simulink model "Controller"  (R2018b)
settings: configuration reference "control_config" (kept outside this file)
values from neighbouring files (symbols this model uses):
  CONTROL_EXPORT = Simulink.Parameter(CONTROL_EXPORT_VALUE)    [controller_model_init.m]
  CONTROL_PARAM = Simulink.Parameter(CONTROL_PARAM_VALUE)    [controller_model_init.m]
undefined symbols (not defined in the file or in its folder): actuator_cmd, CONTROL_CONST, ControlMode, DiscIntNeverNeededParam, timestamp, VehicleStatus
libraries: simulink x21, FMT_Model_Lib x6
settings Model: Creator=jc  LastModifiedBy=jiachi
settings ConfigSetRef: SourceLocation=Base Workspace

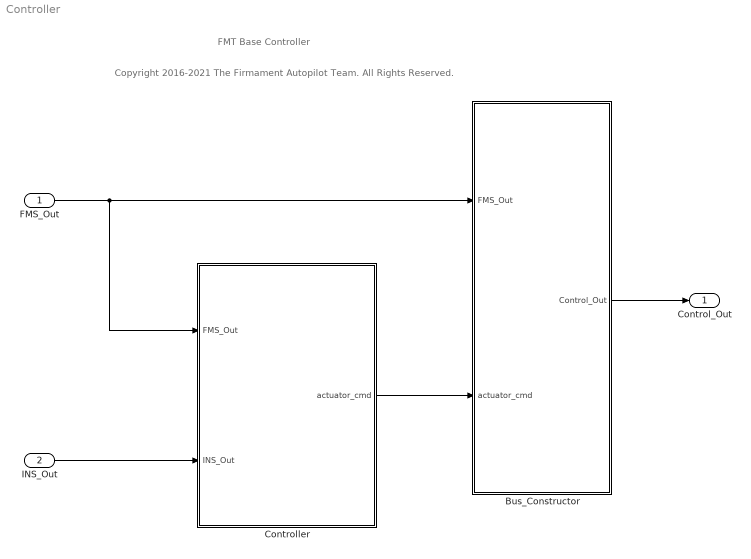
== system Controller ==
  note: Copyright 2016-2021 The Firmament Autopilot Team. All Rights Reserved.
  note: FMT Base Controller
  FMS_Out : Inport  OutDataTypeStr=Bus: FMS_Out_Bus
  INS_Out : Inport  Port=2  OutDataTypeStr=Bus: INS_Out_Bus
  Bus_Constructor : Subsystem
  Controller : Subsystem
  Control_Out : Outport  OutDataTypeStr=Bus: Control_Out_Bus
  wires:
  FMS_Out/1 -> Controller/1(FMS_Out), Bus_Constructor/1(FMS_Out)
  INS_Out/1 -> Controller/2(INS_Out)
  Controller/1(actuator_cmd) -> Bus_Constructor/2(actuator_cmd)
  Bus_Constructor/1(Control_Out) -> Control_Out/1

== system Controller/Bus_Constructor ==
  FMS_Out : Inport
  actuator_cmd : Inport  Port=2
  Bus Assignment : BusAssignment  AssignedSignals=actuator_cmd,timestamp
  Bus Selector : BusSelector  OutputSignals=status
  Bus Selector1 : BusSelector  OutputSignals=actuator_cmd
  Compare To Constant : simulink/Logic and Bit Operations/Compare To Constant  relop===  const=uint8(VehicleStatus.Arm)  OutDataTypeStr=boolean
  Constant : Constant  Value=0  OutDataTypeStr=Bus: Control_Out_Bus
  Switch : Switch  Criteria=u2 > Threshold
  timestamp : Subsystem  mask{sample_time=CONTROL_EXPORT.period}
      mask prompts: sample_time "sample time (ms)"
  Control_Out : Outport
  wires:
  FMS_Out/1 -> Bus Selector1/1, Bus Selector/1
  Bus Selector/1 -> Compare To Constant/1  "<status>"
  Bus Selector1/1 -> Switch/3  "<actuator_cmd>"
  Switch/1 -> Bus Assignment/2
  Compare To Constant/1 -> Switch/2
  actuator_cmd/1 -> Switch/1
  Constant/1 -> Bus Assignment/1
  Bus Assignment/1 -> Control_Out/1
  timestamp/1(timestamp_ms) -> Bus Assignment/3

== system Controller/Controller ==
  FMS_Out : Inport
  INS_Out : Inport  Port=2
  Horizontal_Control : Subsystem
  Static_Control_Allocation : Subsystem
  Vertical_Control : Subsystem
  actuator_cmd : Outport
  wires:
  FMS_Out/1 -> Vertical_Control/1(FMS_Out), Horizontal_Control/1(FMS_Out), Static_Control_Allocation/1(FMS_Out)
  INS_Out/1 -> Horizontal_Control/2(INS_Out), Vertical_Control/2(INS_Out)
  Horizontal_Control/1(rate_dot_cmd_B) -> Static_Control_Allocation/2(rate_dot_cmd_B_normalized)
  Vertical_Control/1(g_force_cmd_B) -> Static_Control_Allocation/3(g_force_cmd_B_normalized)
  Static_Control_Allocation/1(actuator_cmd) -> actuator_cmd/1

== system Controller/Bus_Constructor/timestamp ==
  Constant : Constant  Value=sample_time
  Data Type Conversion : DataTypeConversion  OutDataTypeStr=uint32
  Discrete-Time Integrator : DiscreteIntegrator  IntegratorMethod=Accumulation: Forward Euler  SampleTime=-1  ICPrevOutput=DiscIntNeverNeededParam  ICPrevScaledInput=DiscIntNeverNeededParam
  timestamp_ms : Outport
  wires:
  Discrete-Time Integrator/1 -> Data Type Conversion/1
  Constant/1 -> Discrete-Time Integrator/1
  Data Type Conversion/1 -> timestamp_ms/1

== system Controller/Controller/Horizontal_Control ==
  FMS_Out : Inport
  INS_Out : Inport  Port=2
  Attitude_Controller : Subsystem
  Velocity_Controller : Subsystem
  rate_dot_cmd_B : Outport
  wires:
  Attitude_Controller/1(rate_dot_cmd_B) -> rate_dot_cmd_B/1
  FMS_Out/1 -> Attitude_Controller/2(FMS_Out), Velocity_Controller/1(FMS_Out)
  INS_Out/1 -> Velocity_Controller/2(INS_Out), Attitude_Controller/3(INS_Out)
  Velocity_Controller/1(att_cmd_B_rad) -> Attitude_Controller/1(att_cmd_B_rad)

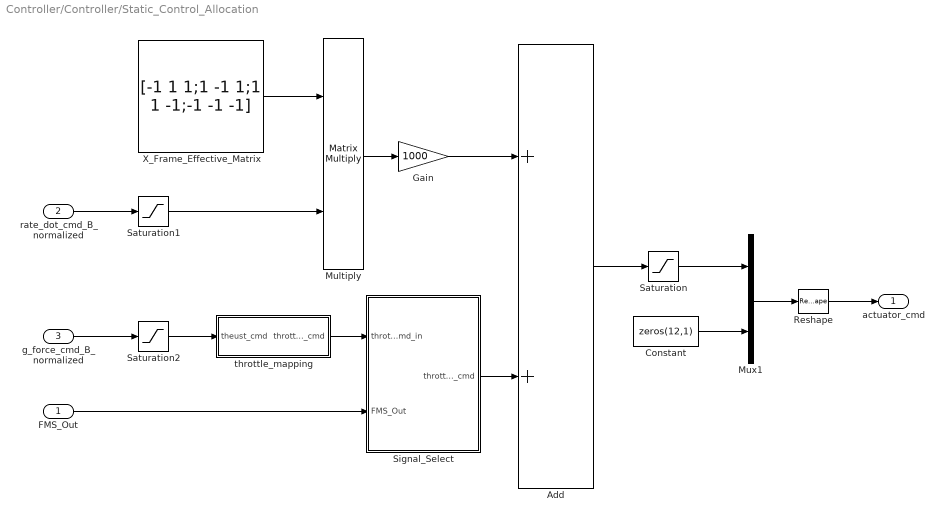
== system Controller/Controller/Static_Control_Allocation ==
  FMS_Out : Inport
  rate_dot_cmd_B_normalized : Inport  Port=2
  g_force_cmd_B_normalized : Inport  Port=3
  Add : Sum  OutDataTypeStr=uint16
  Constant : Constant  Value=zeros(12,1)  VectorParams1D=off  OutDataTypeStr=uint16
  Gain : Gain  Gain=1000  OutDataTypeStr=uint16
  Multiply : Product  Multiplication=Matrix(*)  OutDataTypeStr=Inherit: Same as first input
  Mux1 : Mux  Inputs=2
  Reshape : Reshape  OutputDimensionality=Customize  OutputDimensions=[16,1]
  Saturation : Saturate  UpperLimit=1900  LowerLimit=1100
  Saturation1 : Saturate  UpperLimit=1  LowerLimit=-1
  Saturation2 : Saturate  UpperLimit=1  LowerLimit=-1
  Signal_Select : Subsystem
  X_Frame_Effective_Matrix : Constant  Value=[-1 1 1;1 -1 1;1 1 -1;-1 -1 -1]  OutDataTypeStr=single
  throttle_mapping : Subsystem
  actuator_cmd : Outport
  wires:
  Multiply/1 -> Gain/1
  X_Frame_Effective_Matrix/1 -> Multiply/1
  rate_dot_cmd_B_normalized/1 -> Saturation1/1
  Gain/1 -> Add/1
  g_force_cmd_B_normalized/1 -> Saturation2/1
  Add/1 -> Saturation/1
  Reshape/1 -> actuator_cmd/1
  Mux1/1 -> Reshape/1
  Saturation/1 -> Mux1/1
  Constant/1 -> Mux1/2
  Saturation1/1 -> Multiply/2
  throttle_mapping/1(throttle_cmd) -> Signal_Select/1(throttle_cmd_in)
  Signal_Select/1(throttle_cmd) -> Add/2
  FMS_Out/1 -> Signal_Select/2(FMS_Out)
  Saturation2/1 -> throttle_mapping/1(theust_cmd)

== system Controller/Controller/Vertical_Control ==
  FMS_Out : Inport
  INS_Out : Inport  Port=2
  Veloxity_Z_Controller : Subsystem
  g_force_cmd_B : Outport
  wires:
  INS_Out/1 -> Veloxity_Z_Controller/2(INS_Out)
  Veloxity_Z_Controller/1(g_force_cmd_B) -> g_force_cmd_B/1
  FMS_Out/1 -> Veloxity_Z_Controller/1(FMS_Out)

== system Controller/Controller/Horizontal_Control/Attitude_Controller ==
  att_cmd_B_rad : Inport
  FMS_Out : Inport  Port=2
  INS_Out : Inport  Port=3
  Inner_Loop : Subsystem
  Outter_Loop : Subsystem
  rate_dot_cmd_B : Outport
  wires:
  INS_Out/1 -> Inner_Loop/2(INS_Out), Outter_Loop/2(INS_Out)
  FMS_Out/1 -> Inner_Loop/3(FMS_Out), Outter_Loop/3(FMS_Out)
  att_cmd_B_rad/1 -> Outter_Loop/1(att_cmd_rad)
  Outter_Loop/1(euler_rate_cmd_radPs) -> Inner_Loop/1(euler_rate_cmd_radPs)
  Inner_Loop/1(rate_dot_cmd_B) -> rate_dot_cmd_B/1

== system Controller/Controller/Horizontal_Control/Velocity_Controller ==
  FMS_Out : Inport
  INS_Out : Inport  Port=2
  Accel_to_Attitude_CMD : Subsystem
  Bus Selector : BusSelector  OutputSignals=reset
  Error : Subsystem
  PID_Controller : Subsystem
  Signal_Select : Subsystem
  att_cmd_B_rad : Outport
  wires:
  FMS_Out/1 -> Signal_Select/2(FMS_Out), Error/2(FMS_Out), Bus Selector/1
  PID_Controller/1(accel_cmd_C) -> Signal_Select/1(acc_cmd_in)  "accel_cmd_C_mPs2"
  INS_Out/1 -> Error/1(INS_Out)
  Error/1(uv_err_C_mPs) -> PID_Controller/1(uv_err_C_mPs)
  Accel_to_Attitude_CMD/1(att_cmd_B_rad) -> att_cmd_B_rad/1
  Bus Selector/1 -> PID_Controller/2(reset)  "<reset>"
  Signal_Select/1(acc_cmd_out) -> Accel_to_Attitude_CMD/1(accel_cmd_C_mPs2)

== system Controller/Controller/Static_Control_Allocation/Signal_Select ==
  note: mode:
      | 0: Unknown
      | 1: Mission
      | 2: Position
      | 3: Altitude Hold
      | 4: Manual Mode
      | 5: Acro Mode
  throttle_cmd_in : Inport
  FMS_Out : Inport  Port=2
  Bus Selector1 : BusSelector  OutputSignals=throttle_cmd,ctrl_mode
  Compare To Constant : simulink/Logic and Bit Operations/Compare To Constant  relop===  const=uint8([ControlMode.Manual, ControlMode.Acro, ControlMode.Stabilize])  OutDataTypeStr=boolean
  Compare To Constant1 : simulink/Logic and Bit Operations/Compare To Constant  relop===  const=uint8(ControlMode.Offboard)  OutDataTypeStr=boolean
  Logical Operator : Logic  Operator=OR  Inputs=1  AllPortsSameDT=off  OutDataTypeStr=boolean
  Offboard_Signal_Select : Subsystem
  Switch : Switch  Criteria=u2 > Threshold
  Switch1 : Switch  Criteria=u2 > Threshold
  throttle_cmd : Outport
  wires:
  Compare To Constant/1 -> Logical Operator/1
  FMS_Out/1 -> Offboard_Signal_Select/1(FMS_Out), Bus Selector1/1
  Bus Selector1/1 -> Switch/1  "<throttle_cmd>"
  Bus Selector1/2 -> Compare To Constant1/1, Compare To Constant/1  "<ctrl_mode>"
  Switch/1 -> throttle_cmd/1  "throttle_cmd"
  Logical Operator/1 -> Switch/2
  throttle_cmd_in/1 -> Offboard_Signal_Select/2(throttle_cmd_in), Switch1/3
  Compare To Constant1/1 -> Switch1/2
  Switch1/1 -> Switch/3
  Offboard_Signal_Select/1(throttle_cmd_out) -> Switch1/1

== system Controller/Controller/Static_Control_Allocation/throttle_mapping ==
  theust_cmd : Inport
  Constant1 : Constant  Value=1000  OutDataTypeStr=uint32
  Data Type Conversion : DataTypeConversion  OutDataTypeStr=uint16
  Gain1 : Gain  Gain=1000  OutDataTypeStr=uint32
  Saturation : Saturate  UpperLimit=1  LowerLimit=0
  Sum : Sum  Inputs=|++
  Sum1 : Sum  Inputs=|++
  hover_throttle : Constant  Value=0.5  OutDataTypeStr=Inherit: Inherit via back propagation
  throttle_cmd : Outport
  wires:
  theust_cmd/1 -> Sum/1
  Sum/1 -> Saturation/1
  hover_throttle/1 -> Sum/2
  Gain1/1 -> Sum1/1
  Constant1/1 -> Sum1/2
  Data Type Conversion/1 -> throttle_cmd/1
  Saturation/1 -> Gain1/1
  Sum1/1 -> Data Type Conversion/1

== system Controller/Controller/Vertical_Control/Veloxity_Z_Controller ==
  note: Leave some margin
      | for att control
  FMS_Out : Inport
  INS_Out : Inport  Port=2
  Boosted_Throttle : Subsystem
  Bus Selector : BusSelector  OutputSignals=reset
  Error : Subsystem
  PID_Controller : Subsystem
  Saturation : Saturate  UpperLimit=0.35  LowerLimit=-0.35
  g_force_cmd_B : Outport
  wires:
  Saturation/1 -> g_force_cmd_B/1
  FMS_Out/1 -> Bus Selector/1, Error/1(FMS_Out)
  INS_Out/1 -> Error/2(INS_Out), Boosted_Throttle/2(INS_Out)
  Boosted_Throttle/1(boosted_thrust) -> Saturation/1  "boosted_thrust"
  Error/1(vu_cmd_C_mPs) -> PID_Controller/1(vu_cmd_C_mPs)
  Bus Selector/1 -> PID_Controller/2(reset)  "<reset>"
  PID_Controller/1(thrust_cmd) -> Boosted_Throttle/1(thrust_cmd)

== system Controller/Controller/Horizontal_Control/Attitude_Controller/Inner_Loop ==
  euler_rate_cmd_radPs : Inport
  INS_Out : Inport  Port=2
  FMS_Out : Inport  Port=3
  Bus Selector : BusSelector  OutputSignals=reset
  Rate_Controller : Subsystem
  Signal_Convert : Subsystem
  Signal_Select : Subsystem
  rate_dot_cmd_B : Outport
  wires:
  euler_rate_cmd_radPs/1 -> Signal_Convert/2(euler_rate_cmd)
  Signal_Select/1(out) -> Rate_Controller/1(rate_cmd_radPs)
  Rate_Controller/1(rate_dot_cmd_B) -> rate_dot_cmd_B/1
  Bus Selector/1 -> Rate_Controller/3(reset)  "<reset>"
  INS_Out/1 -> Signal_Convert/3(INS_Out), Rate_Controller/2(INS_Out)
  FMS_Out/1 -> Signal_Convert/1(FMS_Out), Bus Selector/1, Signal_Select/1(FMS_Out)
  Signal_Convert/1(rate_cmd_radPs) -> Signal_Select/2(rate_cmd_radPs)

== system Controller/Controller/Horizontal_Control/Attitude_Controller/Outter_Loop ==
  att_cmd_rad : Inport
  INS_Out : Inport  Port=2
  FMS_Out : Inport  Port=3
  Attitude_Controller : Subsystem
  Signal_Select : Subsystem
  euler_rate_cmd_radPs : Outport
  wires:
  Signal_Select/1(out) -> Attitude_Controller/1(att_cmd_rad)
  FMS_Out/1 -> Signal_Select/2(FMS_Out)
  INS_Out/1 -> Attitude_Controller/2(INS_Out)
  Attitude_Controller/1(euler_rate_cmd_radPs) -> euler_rate_cmd_radPs/1
  att_cmd_rad/1 -> Signal_Select/1(att_cmd_rad)

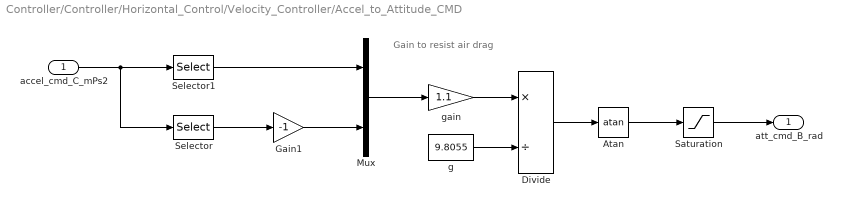
== system Controller/Controller/Horizontal_Control/Velocity_Controller/Accel_to_Attitude_CMD ==
  note: Gain to resist
      | air drag
  accel_cmd_C_mPs2 : Inport
  Atan : Trigonometry  Operator=atan
  Divide : Product  Inputs=*/
  Gain1 : Gain  Gain=-1
  Mux : Mux  Inputs=2
  Saturation : Saturate  UpperLimit=CONTROL_PARAM.ROLL_PITCH_CMD_LIM  LowerLimit=-CONTROL_PARAM.ROLL_PITCH_CMD_LIM
  Selector : Selector  InputPortWidth=2  IndexOptions=Index vector (dialog)  Indices=1  OutputSizes=1
  Selector1 : Selector  InputPortWidth=2  IndexOptions=Index vector (dialog)  Indices=2  OutputSizes=1
  g : Constant  Value=9.8055  OutDataTypeStr=single
  gain : Gain  Gain=1.1
  att_cmd_B_rad : Outport
  wires:
  Mux/1 -> gain/1
  gain/1 -> Divide/1
  Atan/1 -> Saturation/1
  g/1 -> Divide/2
  Divide/1 -> Atan/1
  Selector/1 -> Gain1/1
  Selector1/1 -> Mux/1
  accel_cmd_C_mPs2/1 -> Selector/1, Selector1/1
  Gain1/1 -> Mux/2
  Saturation/1 -> att_cmd_B_rad/1

== system Controller/Controller/Horizontal_Control/Velocity_Controller/Error ==
  INS_Out : Inport
  FMS_Out : Inport  Port=2
  Bus Selector : BusSelector  OutputSignals=u_cmd,v_cmd
  Bus_Select : Subsystem
  Mux : Mux  Inputs=2
  Sum : Sum  Inputs=|+-
  TD : Subsystem
  uv_err_C_mPs : Outport
  wires:
  Sum/1 -> uv_err_C_mPs/1  "uv_error_C_mPs"
  FMS_Out/1 -> Bus Selector/1
  INS_Out/1 -> Bus_Select/1(INS_Out)
  Bus Selector/1 -> Mux/1  "<u_cmd>"
  Bus Selector/2 -> Mux/2  "<v_cmd>"
  Mux/1 -> TD/1(v)
  Bus_Select/1(uv_est_C_mPs) -> Sum/2  "uv_est_C_mPs"
  TD/1(v1) -> Sum/1  "uv_cmd_C_mPs"

== system Controller/Controller/Horizontal_Control/Velocity_Controller/PID_Controller ==
  uv_err_C_mPs : Inport
  reset : Inport  Port=2
  Add : Sum  Inputs=+++
  D_Control : Subsystem  mask{kd=CONTROL_PARAM.VEL_XY_D, max_d=CONTROL_PARAM.VEL_XY_D_MAX, min_d=CONTROL_PARAM.VEL_XY_D_MIN}
  I_Control : Subsystem  mask{ki=CONTROL_PARAM.VEL_XY_I, max_i=CONTROL_PARAM.VEL_XY_I_MAX, min_i=CONTROL_PARAM.VEL_XY_I_MIN}
  P_Control : Subsystem  mask{kp=CONTROL_PARAM.VEL_XY_P}
  accel_cmd_C : Outport
  wires:
  uv_err_C_mPs/1 -> P_Control/1(err), I_Control/1(err), D_Control/1(err)
  reset/1 -> I_Control/2(reset), D_Control/2(reset)
  P_Control/1(p_out) -> Add/1  "accel_p_out"
  I_Control/1(i_out) -> Add/2  "accel_i_out"
  D_Control/1(d_out) -> Add/3  "accel_d_out"
  Add/1 -> accel_cmd_C/1

== system Controller/Controller/Horizontal_Control/Velocity_Controller/Signal_Select ==
  acc_cmd_in : Inport
  FMS_Out : Inport  Port=2
  Bus Selector : BusSelector  OutputSignals=ctrl_mode
  Offboard : simulink/Logic and Bit Operations/Compare To Constant  relop===  const=uint8(ControlMode.Offboard)  OutDataTypeStr=boolean
  Offboard_Signal_Select : Subsystem
  Switch : Switch  Criteria=u2 > Threshold
  acc_cmd_out : Outport
  wires:
  FMS_Out/1 -> Offboard_Signal_Select/1(FMS_Out), Bus Selector/1
  Bus Selector/1 -> Offboard/1  "<ctrl_mode>"
  Offboard/1 -> Switch/2
  Switch/1 -> acc_cmd_out/1
  acc_cmd_in/1 -> Offboard_Signal_Select/2(acc_cmd_in), Switch/3
  Offboard_Signal_Select/1(acc_cmd) -> Switch/1

== system Controller/Controller/Static_Control_Allocation/Signal_Select/Offboard_Signal_Select ==
  FMS_Out : Inport
  throttle_cmd_in : Inport  Port=2
  Bus Selector1 : BusSelector  OutputSignals=cmd_mask
  Bus Selector2 : BusSelector  OutputSignals=throttle_cmd
  Switch : Switch  Criteria=u2 > Threshold
  cmd_throttle valid : simulink/Logic and Bit Operations/Bitwise Operator  logicop=AND  UseBitMask=on  BitMask=bin2dec('1000000000000')  BitMaskRealWorld=Stored Integer
  throttle_cmd_out : Outport
  wires:
  Switch/1 -> throttle_cmd_out/1
  cmd_throttle valid/1 -> Switch/2
  FMS_Out/1 -> Bus Selector2/1, Bus Selector1/1
  Bus Selector1/1 -> cmd_throttle valid/1  "<cmd_mask>"
  Bus Selector2/1 -> Switch/1  "<throttle_cmd>"
  throttle_cmd_in/1 -> Switch/3

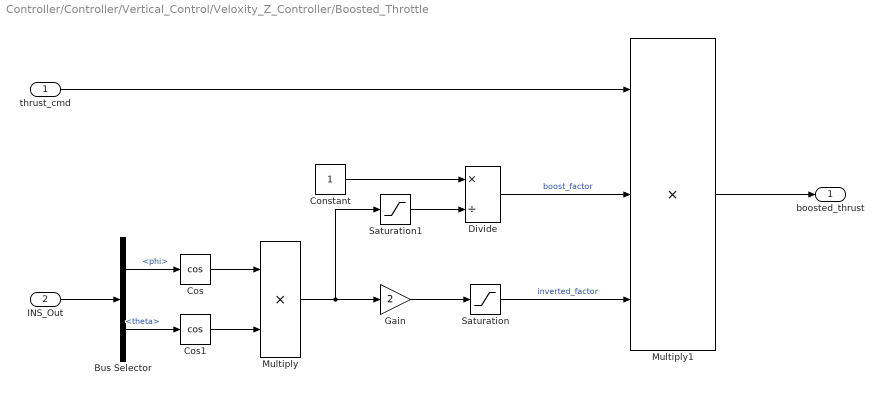
== system Controller/Controller/Vertical_Control/Veloxity_Z_Controller/Boosted_Throttle ==
  thrust_cmd : Inport
  INS_Out : Inport  Port=2
  Bus Selector : BusSelector  OutputSignals=phi,theta
  Constant : Constant  OutDataTypeStr=single
  Cos : Trigonometry  Operator=cos
  Cos1 : Trigonometry  Operator=cos
  Divide : Product  Inputs=*/
  Gain : Gain  Gain=2
  Multiply : Product
  Multiply1 : Product  Inputs=3
  Saturation : Saturate  UpperLimit=1  LowerLimit=0
  Saturation1 : Saturate  UpperLimit=1  LowerLimit=0.5
  boosted_thrust : Outport
  wires:
  INS_Out/1 -> Bus Selector/1
  Bus Selector/1 -> Cos/1  "<phi>"
  Bus Selector/2 -> Cos1/1  "<theta>"
  Cos/1 -> Multiply/1
  Cos1/1 -> Multiply/2
  Multiply/1 -> Saturation1/1, Gain/1
  Gain/1 -> Saturation/1
  Saturation/1 -> Multiply1/3  "inverted_factor"
  Constant/1 -> Divide/1
  Divide/1 -> Multiply1/2  "boost_factor"
  Saturation1/1 -> Divide/2
  thrust_cmd/1 -> Multiply1/1
  Multiply1/1 -> boosted_thrust/1

== system Controller/Controller/Vertical_Control/Veloxity_Z_Controller/Error ==
  FMS_Out : Inport
  INS_Out : Inport  Port=2
  Bus Selector1 : BusSelector  OutputSignals=vd
  Bus Selector2 : BusSelector  OutputSignals=w_cmd
  Gain : Gain  Gain=-1  OutDataTypeStr=Inherit: Same as input
  Signal Copy1 : SignalConversion  OverrideOpt=off
  Sum1 : Sum  Inputs=|+-
  TD : Subsystem
  vu_cmd_C_mPs : Outport
  wires:
  INS_Out/1 -> Bus Selector1/1
  Bus Selector2/1 -> TD/1(v)  "<w_cmd>"
  Bus Selector1/1 -> Signal Copy1/1  "<vd>"
  Gain/1 -> vu_cmd_C_mPs/1
  Sum1/1 -> Gain/1  "w_error_C_mPs"
  FMS_Out/1 -> Bus Selector2/1
  TD/1(v1) -> Sum1/1  "w_cmd_C_mPs"
  Signal Copy1/1 -> Sum1/2  "w_est_C_mPs"

== system Controller/Controller/Vertical_Control/Veloxity_Z_Controller/PID_Controller ==
  vu_cmd_C_mPs : Inport
  reset : Inport  Port=2
  Add : Sum  Inputs=+++
  D_Control : Subsystem  mask{kd=CONTROL_PARAM.VEL_Z_D, max_d=CONTROL_PARAM.VEL_Z_D_MAX, min_d=CONTROL_PARAM.VEL_Z_D_MIN}
  I_Control : Subsystem  mask{ki=CONTROL_PARAM.VEL_Z_I, max_i=CONTROL_PARAM.VEL_Z_I_MAX, min_i=CONTROL_PARAM.VEL_Z_I_MIN}
  P_Control : Subsystem  mask{kp=CONTROL_PARAM.VEL_Z_P}
  thrust_cmd : Outport
  wires:
  P_Control/1(p_out) -> Add/1  "thrust_p_out"
  I_Control/1(i_out) -> Add/2  "thrust_i_out"
  Add/1 -> thrust_cmd/1
  vu_cmd_C_mPs/1 -> D_Control/1(err), I_Control/1(err), P_Control/1(err)
  D_Control/1(d_out) -> Add/3  "thrust_d_out"
  reset/1 -> I_Control/2(reset), D_Control/2(reset)

== system Controller/Controller/Horizontal_Control/Attitude_Controller/Inner_Loop/Rate_Controller ==
  rate_cmd_radPs : Inport
  INS_Out : Inport  Port=2
  reset : Inport  Port=3
  Error : Subsystem
  PID_Controller : Subsystem
  rate_dot_cmd_B : Outport
  wires:
  INS_Out/1 -> Error/2(INS_Out)
  Error/1(rate_err_radPs) -> PID_Controller/1(rate_err_radPs)
  rate_cmd_radPs/1 -> Error/1(rate_cmd_radPs)
  reset/1 -> PID_Controller/2(reset)
  PID_Controller/1(rate_dot_cmd_B) -> rate_dot_cmd_B/1

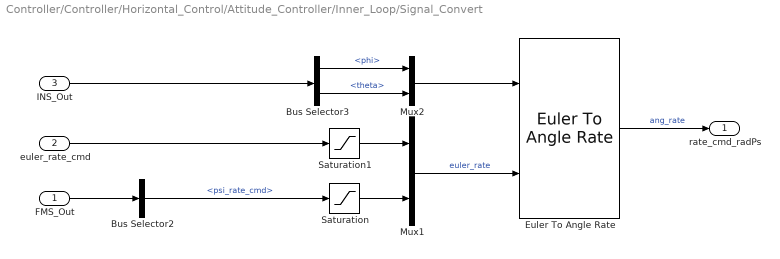
== system Controller/Controller/Horizontal_Control/Attitude_Controller/Inner_Loop/Signal_Convert ==
  FMS_Out : Inport
  euler_rate_cmd : Inport  Port=2
  INS_Out : Inport  Port=3
  Bus Selector2 : BusSelector  OutputSignals=psi_rate_cmd
  Bus Selector3 : BusSelector  OutputSignals=phi,theta
  Euler To Angle Rate : FMT_Model_Lib/Math/Euler To Angle Rate
      settings: SourceProductName=FMT Toolbox
  Mux1 : Mux  Inputs=2
  Mux2 : Mux  Inputs=2
  Saturation : Saturate  UpperLimit=CONTROL_PARAM.R_CMD_LIM  LowerLimit=-CONTROL_PARAM.R_CMD_LIM
  Saturation1 : Saturate  UpperLimit=CONTROL_PARAM.P_Q_CMD_LIM  LowerLimit=-CONTROL_PARAM.P_Q_CMD_LIM
  rate_cmd_radPs : Outport
  wires:
  Bus Selector3/1 -> Mux2/1  "<phi>"
  Mux2/1 -> Euler To Angle Rate/1
  Bus Selector3/2 -> Mux2/2  "<theta>"
  euler_rate_cmd/1 -> Saturation1/1
  Bus Selector2/1 -> Saturation/1  "<psi_rate_cmd>"
  Mux1/1 -> Euler To Angle Rate/2  "euler_rate"
  FMS_Out/1 -> Bus Selector2/1
  INS_Out/1 -> Bus Selector3/1
  Euler To Angle Rate/1 -> rate_cmd_radPs/1  "ang_rate"
  Saturation/1 -> Mux1/2
  Saturation1/1 -> Mux1/1

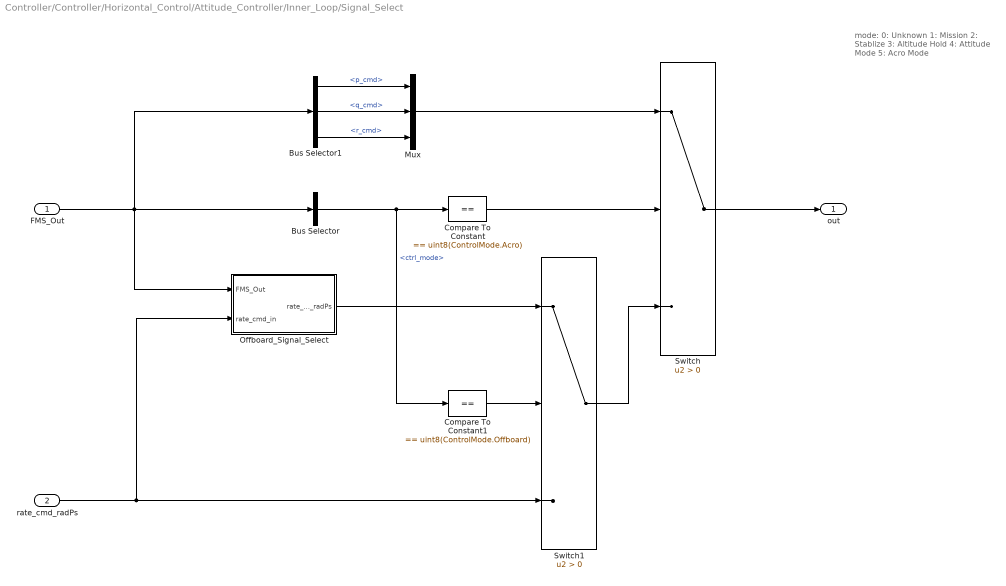
== system Controller/Controller/Horizontal_Control/Attitude_Controller/Inner_Loop/Signal_Select ==
  note: mode:
      | 0: Unknown
      | 1: Mission
      | 2: Stablize
      | 3: Altitude Hold
      | 4: Attitude Mode
      | 5: Acro Mode
  FMS_Out : Inport
  rate_cmd_radPs : Inport  Port=2
  Bus Selector : BusSelector  OutputSignals=ctrl_mode
  Bus Selector1 : BusSelector  OutputSignals=p_cmd,q_cmd,r_cmd
  Compare To Constant : simulink/Logic and Bit Operations/Compare To Constant  relop===  const=uint8(ControlMode.Acro)  OutDataTypeStr=boolean
  Compare To Constant1 : simulink/Logic and Bit Operations/Compare To Constant  relop===  const=uint8(ControlMode.Offboard)  OutDataTypeStr=boolean
  Mux : Mux  Inputs=3
  Offboard_Signal_Select : Subsystem
  Switch : Switch  Criteria=u2 > Threshold
  Switch1 : Switch  Criteria=u2 > Threshold
  out : Outport
  wires:
  FMS_Out/1 -> Bus Selector/1, Offboard_Signal_Select/1(FMS_Out), Bus Selector1/1
  Switch/1 -> out/1
  Bus Selector/1 -> Compare To Constant1/1, Compare To Constant/1  "<ctrl_mode>"
  Compare To Constant/1 -> Switch/2
  Bus Selector1/1 -> Mux/1  "<p_cmd>"
  Bus Selector1/2 -> Mux/2  "<q_cmd>"
  Bus Selector1/3 -> Mux/3  "<r_cmd>"
  Mux/1 -> Switch/1
  rate_cmd_radPs/1 -> Switch1/3, Offboard_Signal_Select/2(rate_cmd_in)
  Switch1/1 -> Switch/3
  Offboard_Signal_Select/1(rate_cmd_radPs) -> Switch1/1
  Compare To Constant1/1 -> Switch1/2

== system Controller/Controller/Horizontal_Control/Attitude_Controller/Outter_Loop/Attitude_Controller ==
  att_cmd_rad : Inport
  INS_Out : Inport  Port=2
  Error : Subsystem
  Sqrt_Root_Controller : Subsystem
  euler_rate_cmd_radPs : Outport
  wires:
  INS_Out/1 -> Error/2(INS_Out)
  Sqrt_Root_Controller/1(euler_rate_cmd_radPs) -> euler_rate_cmd_radPs/1
  att_cmd_rad/1 -> Error/1(att_cmd)
  Error/1(euler_err_rad) -> Sqrt_Root_Controller/1(euler_err_rad)

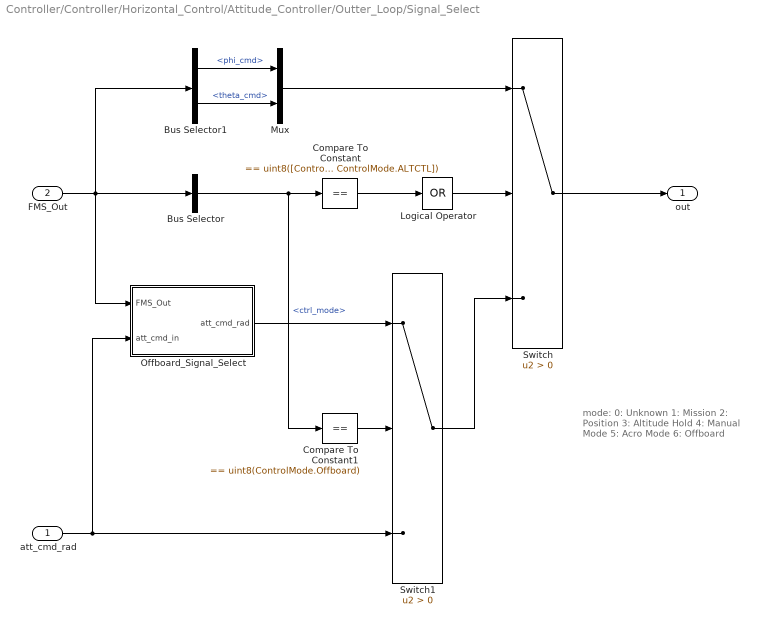
== system Controller/Controller/Horizontal_Control/Attitude_Controller/Outter_Loop/Signal_Select ==
  note: mode:
      | 0: Unknown
      | 1: Mission
      | 2: Position
      | 3: Altitude Hold
      | 4: Manual Mode
      | 5: Acro Mode
      | 6: Offboard
  att_cmd_rad : Inport
  FMS_Out : Inport  Port=2
  Bus Selector : BusSelector  OutputSignals=ctrl_mode
  Bus Selector1 : BusSelector  OutputSignals=phi_cmd,theta_cmd
  Compare To Constant : simulink/Logic and Bit Operations/Compare To Constant  relop===  const=uint8([ControlMode.Stabilize, ControlMode.ALTCTL])  OutDataTypeStr=boolean
  Compare To Constant1 : simulink/Logic and Bit Operations/Compare To Constant  relop===  const=uint8(ControlMode.Offboard)  OutDataTypeStr=boolean
  Logical Operator : Logic  Operator=OR  Inputs=1  AllPortsSameDT=off  OutDataTypeStr=boolean
  Mux : Mux  Inputs=2
  Offboard_Signal_Select : Subsystem
  Switch : Switch  Criteria=u2 > Threshold
  Switch1 : Switch  Criteria=u2 > Threshold
  out : Outport
  wires:
  Compare To Constant/1 -> Logical Operator/1
  Bus Selector1/2 -> Mux/2  "<theta_cmd>"
  Bus Selector1/1 -> Mux/1  "<phi_cmd>"
  Bus Selector/1 -> Compare To Constant1/1, Compare To Constant/1  "<ctrl_mode>"
  FMS_Out/1 -> Bus Selector/1, Bus Selector1/1, Offboard_Signal_Select/1(FMS_Out)
  Mux/1 -> Switch/1
  Switch/1 -> out/1
  Logical Operator/1 -> Switch/2
  Switch1/1 -> Switch/3
  Compare To Constant1/1 -> Switch1/2
  Offboard_Signal_Select/1(att_cmd_rad) -> Switch1/1
  att_cmd_rad/1 -> Offboard_Signal_Select/2(att_cmd_in), Switch1/3

== system Controller/Controller/Horizontal_Control/Velocity_Controller/Error/Bus_Select ==
  INS_Out : Inport
  Bus Selector1 : BusSelector  OutputSignals=vn,ve
  Bus Selector2 : BusSelector  OutputSignals=psi
  Constant : Constant  Value=0  OutDataTypeStr=single
  Multiply : Product  Multiplication=Matrix(*)
  Mux2 : Mux  Inputs=3
  Psi To DCM : FMT_Model_Lib/Transformation/Psi To DCM
      settings: SourceProductName=FMT Toolbox
  Selector : Selector  InputPortWidth=3  IndexOptions=Index vector (dialog)  Indices=[1 2]  OutputSizes=1
  uv_est_C_mPs : Outport
  wires:
  Psi To DCM/1 -> Multiply/1
  Bus Selector2/1 -> Psi To DCM/1  "<psi>"
  Constant/1 -> Mux2/3  "<velD>"
  Mux2/1 -> Multiply/2
  Bus Selector1/2 -> Mux2/2  "<ve>"
  Bus Selector1/1 -> Mux2/1  "<vn>"
  INS_Out/1 -> Bus Selector2/1, Bus Selector1/1
  Multiply/1 -> Selector/1
  Selector/1 -> uv_est_C_mPs/1

== system Controller/Controller/Horizontal_Control/Velocity_Controller/Error/TD ==
  v : Inport
  Integrator : DiscreteIntegrator  SampleTime=-1  ICPrevOutput=DiscIntNeverNeededParam  ICPrevScaledInput=DiscIntNeverNeededParam
  Integrator1 : DiscreteIntegrator  SampleTime=-1  ICPrevOutput=DiscIntNeverNeededParam  ICPrevScaledInput=DiscIntNeverNeededParam
  Subtract : Sum  Inputs=+-
  "fhan " : Subsystem  mask{r0=6*9.806, h0=0.05}
      mask DialogControl ParameterGroupVar Prompt: fhan(v1,v2,r0,h0)
  v1 : Outport
  wires:
  Integrator1/1 -> v1/1, Subtract/1
  v/1 -> Subtract/2
  Integrator/1 -> "fhan "/2(v2), Integrator1/1  "v2"
  Subtract/1 -> "fhan "/1(v1)
  "fhan "/1(fhan) -> Integrator/1

== system Controller/Controller/Horizontal_Control/Velocity_Controller/PID_Controller/D_Control ==
  err : Inport
  reset : Inport  Port=2
  DT Filter : FMT_Model_Lib/Filter/DT Filter  fc=10
      settings: SourceProductName=FMT Toolbox
  Multiply : Product  OutDataTypeStr=Inherit: Same as first input
  Saturation : Saturate  UpperLimit=max_d  LowerLimit=min_d
  kd : Constant  Value=kd  OutDataTypeStr=single
  d_out : Outport
  wires:
  err/1 -> DT Filter/1
  kd/1 -> Multiply/1
  Multiply/1 -> Saturation/1
  Saturation/1 -> d_out/1
  reset/1 -> DT Filter/2
  DT Filter/1 -> Multiply/2

== system Controller/Controller/Horizontal_Control/Velocity_Controller/PID_Controller/I_Control ==
  err : Inport
  reset : Inport  Port=2
  Constant : Constant  Value=0  OutDataTypeStr=single
  Discrete-Time Integrator : DiscreteIntegrator  ExternalReset=level  InitialConditionSource=external  SampleTime=-1  LimitOutput=on  UpperSaturationLimit=max_i  LowerSaturationLimit=min_i  ICPrevOutput=DiscIntNeverNeededParam  ICPrevScaledInput=DiscIntNeverNeededParam
  Multiply : Product  OutDataTypeStr=Inherit: Same as first input
  ki : Constant  Value=ki  OutDataTypeStr=single
  i_out : Outport
  wires:
  err/1 -> Multiply/2
  Multiply/1 -> Discrete-Time Integrator/1
  reset/1 -> Discrete-Time Integrator/2
  Constant/1 -> Discrete-Time Integrator/3
  Discrete-Time Integrator/1 -> i_out/1
  ki/1 -> Multiply/1

== system Controller/Controller/Horizontal_Control/Velocity_Controller/PID_Controller/P_Control ==
  err : Inport
  Multiply : Product  OutDataTypeStr=Inherit: Same as first input
  kp : Constant  Value=kp  OutDataTypeStr=single
  p_out : Outport
  wires:
  err/1 -> Multiply/2
  kp/1 -> Multiply/1
  Multiply/1 -> p_out/1

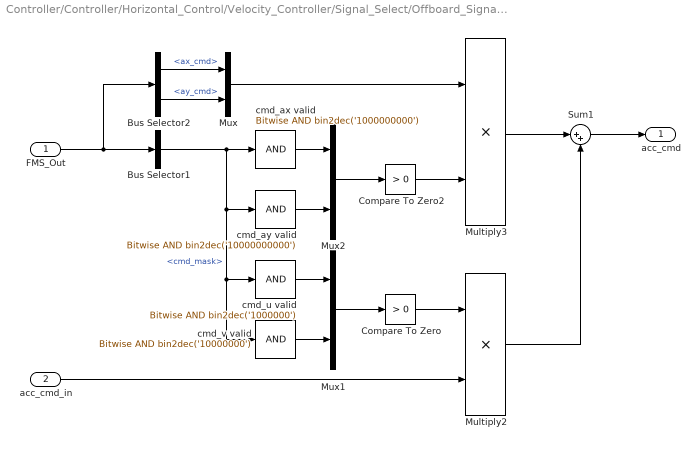
== system Controller/Controller/Horizontal_Control/Velocity_Controller/Signal_Select/Offboard_Signal_Select ==
  FMS_Out : Inport
  acc_cmd_in : Inport  Port=2
  Bus Selector1 : BusSelector  OutputSignals=cmd_mask
  Bus Selector2 : BusSelector  OutputSignals=ax_cmd,ay_cmd
  Compare To Zero : simulink/Logic and Bit Operations/Compare To Zero  relop=>  OutDataTypeStr=boolean
  Compare To Zero2 : simulink/Logic and Bit Operations/Compare To Zero  relop=>  OutDataTypeStr=boolean
  Multiply2 : Product
  Multiply3 : Product
  Mux : Mux  Inputs=2
  Mux1 : Mux  Inputs=2
  Mux2 : Mux  Inputs=2
  Sum1 : Sum  Inputs=|++
  cmd_ax valid : simulink/Logic and Bit Operations/Bitwise Operator  logicop=AND  UseBitMask=on  BitMask=bin2dec('1000000000')  BitMaskRealWorld=Stored Integer
  cmd_ay valid : simulink/Logic and Bit Operations/Bitwise Operator  logicop=AND  UseBitMask=on  BitMask=bin2dec('10000000000')  BitMaskRealWorld=Stored Integer
  cmd_u valid : simulink/Logic and Bit Operations/Bitwise Operator  logicop=AND  UseBitMask=on  BitMask=bin2dec('1000000')  BitMaskRealWorld=Stored Integer
  cmd_v valid : simulink/Logic and Bit Operations/Bitwise Operator  logicop=AND  UseBitMask=on  BitMask=bin2dec('10000000')  BitMaskRealWorld=Stored Integer
  acc_cmd : Outport
  wires:
  Multiply2/1 -> Sum1/2
  FMS_Out/1 -> Bus Selector2/1, Bus Selector1/1
  Bus Selector1/1 -> cmd_v valid/1, cmd_u valid/1, cmd_ay valid/1, cmd_ax valid/1  "<cmd_mask>"
  Multiply3/1 -> Sum1/1
  cmd_u valid/1 -> Mux1/1
  cmd_v valid/1 -> Mux1/2
  Mux1/1 -> Compare To Zero/1
  acc_cmd_in/1 -> Multiply2/2
  Compare To Zero/1 -> Multiply2/1
  Bus Selector2/1 -> Mux/1  "<ax_cmd>"
  cmd_ax valid/1 -> Mux2/1
  cmd_ay valid/1 -> Mux2/2
  Mux2/1 -> Compare To Zero2/1
  Compare To Zero2/1 -> Multiply3/2
  Bus Selector2/2 -> Mux/2  "<ay_cmd>"
  Mux/1 -> Multiply3/1
  Sum1/1 -> acc_cmd/1

== system Controller/Controller/Vertical_Control/Veloxity_Z_Controller/Error/TD ==
  v : Inport
  Integrator : DiscreteIntegrator  SampleTime=-1  ICPrevOutput=DiscIntNeverNeededParam  ICPrevScaledInput=DiscIntNeverNeededParam
  Integrator1 : DiscreteIntegrator  SampleTime=-1  ICPrevOutput=DiscIntNeverNeededParam  ICPrevScaledInput=DiscIntNeverNeededParam
  Subtract : Sum  Inputs=+-
  "fhan " : Subsystem  mask{r0=8*9.806, h0=0.05}
      mask DialogControl ParameterGroupVar Prompt: fhan(v1,v2,r0,h0)
  v1 : Outport
  wires:
  Integrator1/1 -> v1/1, Subtract/1
  v/1 -> Subtract/2
  Integrator/1 -> "fhan "/2(v2), Integrator1/1  "v2"
  Subtract/1 -> "fhan "/1(v1)
  "fhan "/1(fhan) -> Integrator/1

== system Controller/Controller/Vertical_Control/Veloxity_Z_Controller/PID_Controller/D_Control ==
  err : Inport
  reset : Inport  Port=2
  DT Filter : FMT_Model_Lib/Filter/DT Filter  fc=10
      settings: SourceProductName=FMT Toolbox
  Multiply : Product  OutDataTypeStr=Inherit: Same as first input
  Saturation : Saturate  UpperLimit=max_d  LowerLimit=min_d
  kd : Constant  Value=kd  OutDataTypeStr=single
  d_out : Outport
  wires:
  err/1 -> DT Filter/1
  kd/1 -> Multiply/1
  Multiply/1 -> Saturation/1
  Saturation/1 -> d_out/1
  reset/1 -> DT Filter/2
  DT Filter/1 -> Multiply/2

== system Controller/Controller/Vertical_Control/Veloxity_Z_Controller/PID_Controller/I_Control ==
  err : Inport
  reset : Inport  Port=2
  Constant : Constant  Value=0  OutDataTypeStr=single
  Discrete-Time Integrator : DiscreteIntegrator  ExternalReset=level  InitialConditionSource=external  SampleTime=-1  LimitOutput=on  UpperSaturationLimit=max_i  LowerSaturationLimit=min_i  ICPrevOutput=DiscIntNeverNeededParam  ICPrevScaledInput=DiscIntNeverNeededParam
  Multiply : Product  OutDataTypeStr=Inherit: Same as first input
  ki : Constant  Value=ki  OutDataTypeStr=single
  i_out : Outport
  wires:
  err/1 -> Multiply/2
  Multiply/1 -> Discrete-Time Integrator/1
  reset/1 -> Discrete-Time Integrator/2
  Constant/1 -> Discrete-Time Integrator/3
  Discrete-Time Integrator/1 -> i_out/1
  ki/1 -> Multiply/1

== system Controller/Controller/Vertical_Control/Veloxity_Z_Controller/PID_Controller/P_Control ==
  err : Inport
  Multiply : Product  OutDataTypeStr=Inherit: Same as first input
  kp : Constant  Value=kp  OutDataTypeStr=single
  p_out : Outport
  wires:
  err/1 -> Multiply/2
  kp/1 -> Multiply/1
  Multiply/1 -> p_out/1

== system Controller/Controller/Horizontal_Control/Attitude_Controller/Inner_Loop/Rate_Controller/Error ==
  rate_cmd_radPs : Inport
  INS_Out : Inport  Port=2
  Bus_Select : Subsystem
  First Order LPF : FMT_Model_Lib/Filter/First Order LPF  fc=30
      settings: SourceProductName=FMT Toolbox
  Sum : Sum  Inputs=|+-
  rate_err_radPs : Outport
  wires:
  Sum/1 -> First Order LPF/1  "rate_error_B_radPs"
  rate_cmd_radPs/1 -> Sum/1  "rate_cmd_B_radPs"
  INS_Out/1 -> Bus_Select/1(INS_Out)
  Bus_Select/1(rate_est_radPs) -> Sum/2  "rate_est_B_radPs"
  First Order LPF/1 -> rate_err_radPs/1

== system Controller/Controller/Horizontal_Control/Attitude_Controller/Inner_Loop/Rate_Controller/PID_Controller ==
  rate_err_radPs : Inport
  reset : Inport  Port=2
  Add : Sum  Inputs=+++
  D_Control : Subsystem  mask{p_kd=CONTROL_PARAM.ROLL_RATE_D, q_kd=CONTROL_PARAM.PITCH_RATE_D, r_kd=CONTROL_PARAM.YAW_RATE_D, max_d=CONTROL_PARAM.RATE_D_MAX, min_d=CONTROL_PARAM.RATE_D_MIN}
  I_Control : Subsystem  mask{p_ki=CONTROL_PARAM.ROLL_RATE_I, q_ki=CONTROL_PARAM.PITCH_RATE_I, r_ki=CONTROL_PARAM.YAW_RATE_I, max_i=CONTROL_PARAM.RATE_I_MAX, min_i=CONTROL_PARAM.RATE_I_MIN}
  P_Control : Subsystem  mask{p_kp=CONTROL_PARAM.ROLL_RATE_P, q_kp=CONTROL_PARAM.PITCH_RATE_P, r_kp=CONTROL_PARAM.YAW_RATE_P}
  rate_dot_cmd_B : Outport
  wires:
  rate_err_radPs/1 -> P_Control/1(err), I_Control/1(err), D_Control/1(err)
  P_Control/1(p_out) -> Add/1  "torque_p_out"
  I_Control/1(i_out) -> Add/2  "torque_i_out"
  D_Control/1(d_out) -> Add/3  "torque_d_out"
  reset/1 -> I_Control/2(reset), D_Control/2(reset)
  Add/1 -> rate_dot_cmd_B/1

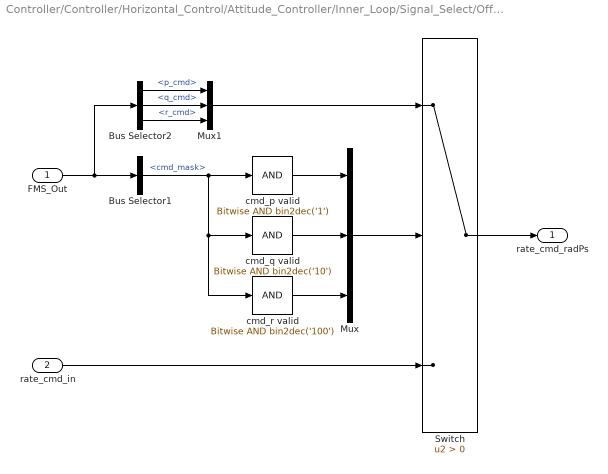
== system Controller/Controller/Horizontal_Control/Attitude_Controller/Inner_Loop/Signal_Select/Offboard_Signal_Select ==
  FMS_Out : Inport
  rate_cmd_in : Inport  Port=2
  Bus Selector1 : BusSelector  OutputSignals=cmd_mask
  Bus Selector2 : BusSelector  OutputSignals=p_cmd,q_cmd,r_cmd
  Mux : Mux  Inputs=3
  Mux1 : Mux  Inputs=3
  Switch : Switch  Criteria=u2 > Threshold
  cmd_p valid : simulink/Logic and Bit Operations/Bitwise Operator  logicop=AND  UseBitMask=on  BitMask=bin2dec('1')  BitMaskRealWorld=Stored Integer
  cmd_q valid : simulink/Logic and Bit Operations/Bitwise Operator  logicop=AND  UseBitMask=on  BitMask=bin2dec('10')  BitMaskRealWorld=Stored Integer
  cmd_r valid : simulink/Logic and Bit Operations/Bitwise Operator  logicop=AND  UseBitMask=on  BitMask=bin2dec('100')  BitMaskRealWorld=Stored Integer
  rate_cmd_radPs : Outport
  wires:
  FMS_Out/1 -> Bus Selector2/1, Bus Selector1/1
  Bus Selector1/1 -> cmd_r valid/1, cmd_q valid/1, cmd_p valid/1  "<cmd_mask>"
  rate_cmd_in/1 -> Switch/3
  Switch/1 -> rate_cmd_radPs/1
  cmd_p valid/1 -> Mux/1
  cmd_q valid/1 -> Mux/2
  cmd_r valid/1 -> Mux/3
  Mux/1 -> Switch/2
  Bus Selector2/1 -> Mux1/1  "<p_cmd>"
  Bus Selector2/2 -> Mux1/2  "<q_cmd>"
  Bus Selector2/3 -> Mux1/3  "<r_cmd>"
  Mux1/1 -> Switch/1

== system Controller/Controller/Horizontal_Control/Attitude_Controller/Outter_Loop/Attitude_Controller/Error ==
  att_cmd : Inport
  INS_Out : Inport  Port=2
  Bus_Select : Subsystem
  Sum : Sum  Inputs=|+-
  euler_err_rad : Outport
  wires:
  att_cmd/1 -> Sum/1  "att_cmd_B_rad"
  Sum/1 -> euler_err_rad/1  "att_error_B_rad"
  INS_Out/1 -> Bus_Select/1(INS_Out)
  Bus_Select/1(att_est_B_rad) -> Sum/2  "att_est_B_rad"

== system Controller/Controller/Horizontal_Control/Attitude_Controller/Outter_Loop/Attitude_Controller/Sqrt_Root_Controller ==
  euler_err_rad : Inport
  Constant1 : Constant  Value=CONTROL_PARAM.ROLL_P
  Constant2 : Constant  Value=CONTROL_PARAM.PITCH_P
  Mux : Mux  Inputs=2
  Sqrt_Root_Control : Subsystem  mask{dt=CONTROL_CONST.dt, second_ord_lim=9.5993}
      mask prompts: second_ord_lim "2nd-order lim"
  euler_rate_cmd_radPs : Outport
  wires:
  Sqrt_Root_Control/1(out) -> euler_rate_cmd_radPs/1
  euler_err_rad/1 -> Sqrt_Root_Control/1(error)
  Mux/1 -> Sqrt_Root_Control/2(p)
  Constant1/1 -> Mux/1
  Constant2/1 -> Mux/2

== system Controller/Controller/Horizontal_Control/Attitude_Controller/Outter_Loop/Signal_Select/Offboard_Signal_Select ==
  FMS_Out : Inport
  att_cmd_in : Inport  Port=2
  Bus Selector1 : BusSelector  OutputSignals=cmd_mask
  Bus Selector2 : BusSelector  OutputSignals=phi_cmd,theta_cmd
  Mux1 : Mux  Inputs=2
  Mux2 : Mux  Inputs=2
  Switch : Switch  Criteria=u2 > Threshold
  cmd_phi valid : simulink/Logic and Bit Operations/Bitwise Operator  logicop=AND  UseBitMask=on  BitMask=bin2dec('1000')  BitMaskRealWorld=Stored Integer
  cmd_theta valid : simulink/Logic and Bit Operations/Bitwise Operator  logicop=AND  UseBitMask=on  BitMask=bin2dec('10000')  BitMaskRealWorld=Stored Integer
  att_cmd_rad : Outport
  wires:
  Switch/1 -> att_cmd_rad/1
  FMS_Out/1 -> Bus Selector2/1, Bus Selector1/1
  Bus Selector1/1 -> cmd_theta valid/1, cmd_phi valid/1  "<cmd_mask>"
  cmd_phi valid/1 -> Mux1/1
  cmd_theta valid/1 -> Mux1/2
  Mux1/1 -> Switch/2
  Bus Selector2/1 -> Mux2/1  "<phi_cmd>"
  Bus Selector2/2 -> Mux2/2  "<theta_cmd>"
  Mux2/1 -> Switch/1
  att_cmd_in/1 -> Switch/3

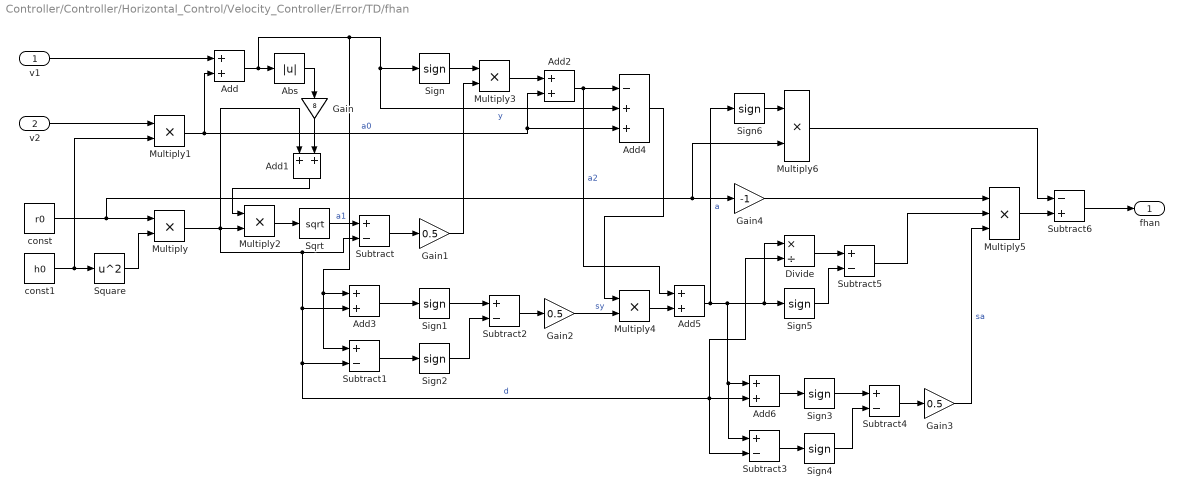
== system Controller/Controller/Horizontal_Control/Velocity_Controller/Error/TD/fhan  ==
  v1 : Inport
  v2 : Inport  Port=2
  Abs : Abs
  Add{,1..3,5..6} (6 alike) : Sum  OutDataTypeStr=Inherit: Same as first input
  Add4 : Sum  Inputs=-++
  Divide : Product  Inputs=*/
  Gain : Gain  Gain=8
  Gain1 : Gain  Gain=0.5  OutDataTypeStr=Inherit: Same as input
  Gain2 : Gain  Gain=0.5  OutDataTypeStr=Inherit: Same as input
  Gain3 : Gain  Gain=0.5  OutDataTypeStr=Inherit: Same as input
  Gain4 : Gain  Gain=-1  OutDataTypeStr=Inherit: Same as input
  Multiply{,1..3} (4 alike) : Product  OutDataTypeStr=Inherit: Same as first input
  Multiply4 : Product  OutDataTypeStr=single
  Multiply5 : Product  Inputs=3
  Multiply6 : Product  OutDataTypeStr=single
  Sign{,1..6} (7 alike) : Signum
  Sqrt : Sqrt  SaturateOnIntegerOverflow=on
  Square : Math  Operator=square  SaturateOnIntegerOverflow=on
  Subtract{,1..5} (6 alike) : Sum  Inputs=+-  OutDataTypeStr=Inherit: Same as first input
  Subtract6 : Sum  Inputs=-+  OutDataTypeStr=Inherit: Same as first input
  const : Constant  Value=r0  OutDataTypeStr=single
  const1 : Constant  Value=h0  OutDataTypeStr=single
  fhan : Outport
  wires:
  Sign1/1 -> Subtract2/1
  Multiply2/1 -> Sqrt/1
  Square/1 -> Multiply/2
  Gain1/1 -> Multiply3/2
  Multiply6/1 -> Subtract6/1
  Multiply/1 -> Multiply2/2, Add1/1, Add3/2, Subtract1/2, Add6/2, Subtract3/2, Divide/2, Subtract/2  "d"
  Add6/1 -> Sign3/1
  Sign3/1 -> Subtract4/1
  Sign6/1 -> Multiply6/1
  Multiply5/1 -> Subtract6/2
  Gain4/1 -> Multiply5/1
  Subtract4/1 -> Gain3/1
  Add2/1 -> Add5/1, Add4/1  "a2"
  Subtract2/1 -> Gain2/1
  Add/1 -> Abs/1, Sign/1, Add4/2, Add3/1, Subtract1/1  "y"
  Multiply1/1 -> Add/2, Add2/2, Add4/3  "a0"
  Add5/1 -> Add6/1, Subtract3/1, Divide/1, Sign5/1, Sign6/1  "a"
  const1/1 -> Square/1, Multiply1/2
  Multiply4/1 -> Add5/2
  Subtract5/1 -> Multiply5/2
  Add3/1 -> Sign1/1
  const/1 -> Multiply/1, Gain4/1, Multiply6/2
  Gain/1 -> Add1/2
  Multiply3/1 -> Add2/1
  Divide/1 -> Subtract5/1
  Subtract1/1 -> Sign2/1
  Add1/1 -> Multiply2/1
  Subtract3/1 -> Sign4/1
  Sqrt/1 -> Subtract/1  "a1"
  Sign5/1 -> Subtract5/2
  Add4/1 -> Multiply4/1
  Abs/1 -> Gain/1
  Sign4/1 -> Subtract4/2
  Sign2/1 -> Subtract2/2
  Subtract6/1 -> fhan/1
  Subtract/1 -> Gain1/1
  Gain3/1 -> Multiply5/3  "sa"
  v2/1 -> Multiply1/1
  Gain2/1 -> Multiply4/2  "sy"
  Sign/1 -> Multiply3/1
  v1/1 -> Add/1

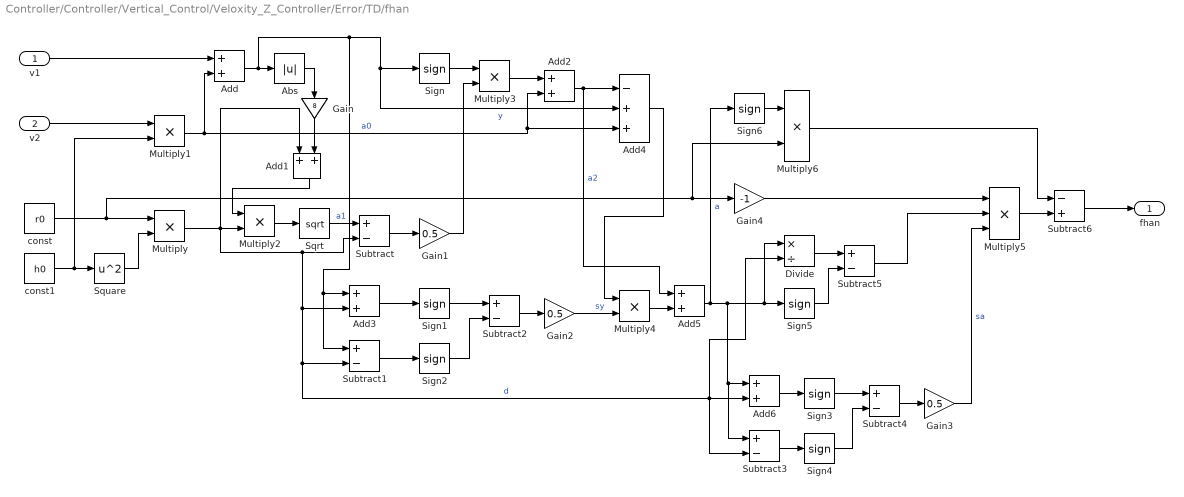
== system Controller/Controller/Vertical_Control/Veloxity_Z_Controller/Error/TD/fhan  ==
  v1 : Inport
  v2 : Inport  Port=2
  Abs : Abs
  Add{,1..3,5..6} (6 alike) : Sum  OutDataTypeStr=Inherit: Same as first input
  Add4 : Sum  Inputs=-++
  Divide : Product  Inputs=*/
  Gain : Gain  Gain=8
  Gain1 : Gain  Gain=0.5  OutDataTypeStr=Inherit: Same as input
  Gain2 : Gain  Gain=0.5  OutDataTypeStr=Inherit: Same as input
  Gain3 : Gain  Gain=0.5  OutDataTypeStr=Inherit: Same as input
  Gain4 : Gain  Gain=-1  OutDataTypeStr=Inherit: Same as input
  Multiply{,1..3} (4 alike) : Product  OutDataTypeStr=Inherit: Same as first input
  Multiply4 : Product  OutDataTypeStr=single
  Multiply5 : Product  Inputs=3
  Multiply6 : Product  OutDataTypeStr=single
  Sign{,1..6} (7 alike) : Signum
  Sqrt : Sqrt  SaturateOnIntegerOverflow=on
  Square : Math  Operator=square  SaturateOnIntegerOverflow=on
  Subtract{,1..5} (6 alike) : Sum  Inputs=+-  OutDataTypeStr=Inherit: Same as first input
  Subtract6 : Sum  Inputs=-+  OutDataTypeStr=Inherit: Same as first input
  const : Constant  Value=r0  OutDataTypeStr=single
  const1 : Constant  Value=h0  OutDataTypeStr=single
  fhan : Outport
  wires:
  Sign1/1 -> Subtract2/1
  Multiply2/1 -> Sqrt/1
  Square/1 -> Multiply/2
  Gain1/1 -> Multiply3/2
  Multiply6/1 -> Subtract6/1
  Multiply/1 -> Multiply2/2, Add1/1, Add3/2, Subtract1/2, Add6/2, Subtract3/2, Divide/2, Subtract/2  "d"
  Add6/1 -> Sign3/1
  Sign3/1 -> Subtract4/1
  Sign6/1 -> Multiply6/1
  Multiply5/1 -> Subtract6/2
  Gain4/1 -> Multiply5/1
  Subtract4/1 -> Gain3/1
  Add2/1 -> Add5/1, Add4/1  "a2"
  Subtract2/1 -> Gain2/1
  Add/1 -> Abs/1, Sign/1, Add4/2, Add3/1, Subtract1/1  "y"
  Multiply1/1 -> Add/2, Add2/2, Add4/3  "a0"
  Add5/1 -> Add6/1, Subtract3/1, Divide/1, Sign5/1, Sign6/1  "a"
  const1/1 -> Square/1, Multiply1/2
  Multiply4/1 -> Add5/2
  Subtract5/1 -> Multiply5/2
  Add3/1 -> Sign1/1
  const/1 -> Multiply/1, Gain4/1, Multiply6/2
  Gain/1 -> Add1/2
  Multiply3/1 -> Add2/1
  Divide/1 -> Subtract5/1
  Subtract1/1 -> Sign2/1
  Add1/1 -> Multiply2/1
  Subtract3/1 -> Sign4/1
  Sqrt/1 -> Subtract/1  "a1"
  Sign5/1 -> Subtract5/2
  Add4/1 -> Multiply4/1
  Abs/1 -> Gain/1
  Sign4/1 -> Subtract4/2
  Sign2/1 -> Subtract2/2
  Subtract6/1 -> fhan/1
  Subtract/1 -> Gain1/1
  Gain3/1 -> Multiply5/3  "sa"
  v2/1 -> Multiply1/1
  Gain2/1 -> Multiply4/2  "sy"
  Sign/1 -> Multiply3/1
  v1/1 -> Add/1

== system Controller/Controller/Horizontal_Control/Attitude_Controller/Inner_Loop/Rate_Controller/Error/Bus_Select ==
  INS_Out : Inport
  Bus Selector1 : BusSelector  OutputSignals=p,q,r
  Mux1 : Mux  Inputs=3
  rate_est_radPs : Outport
  wires:
  Bus Selector1/1 -> Mux1/1  "<p>"
  Bus Selector1/3 -> Mux1/3  "<r>"
  Bus Selector1/2 -> Mux1/2  "<q>"
  Mux1/1 -> rate_est_radPs/1
  INS_Out/1 -> Bus Selector1/1

== system Controller/Controller/Horizontal_Control/Attitude_Controller/Inner_Loop/Rate_Controller/PID_Controller/D_Control ==
  err : Inport
  reset : Inport  Port=2
  DT Filter : FMT_Model_Lib/Filter/DT Filter  fc=30
      settings: SourceProductName=FMT Toolbox
  Multiply : Product  OutDataTypeStr=Inherit: Same as first input
  Mux : Mux  Inputs=3
  Saturation : Saturate  UpperLimit=max_d  LowerLimit=min_d
  gain1 : Constant  Value=p_kd  OutDataTypeStr=single
  gain2 : Constant  Value=q_kd  OutDataTypeStr=single
  gain3 : Constant  Value=r_kd  OutDataTypeStr=single
  d_out : Outport
  wires:
  err/1 -> DT Filter/1
  gain2/1 -> Mux/2
  gain1/1 -> Mux/1
  Multiply/1 -> Saturation/1
  gain3/1 -> Mux/3
  Saturation/1 -> d_out/1
  reset/1 -> DT Filter/2
  Mux/1 -> Multiply/1
  DT Filter/1 -> Multiply/2

== system Controller/Controller/Horizontal_Control/Attitude_Controller/Inner_Loop/Rate_Controller/PID_Controller/I_Control ==
  err : Inport
  reset : Inport  Port=2
  Constant : Constant  Value=[0;0;0]  OutDataTypeStr=single
  Discrete-Time Integrator : DiscreteIntegrator  ExternalReset=level  InitialConditionSource=external  SampleTime=-1  LimitOutput=on  UpperSaturationLimit=max_i  LowerSaturationLimit=min_i  ICPrevOutput=DiscIntNeverNeededParam  ICPrevScaledInput=DiscIntNeverNeededParam
  Multiply : Product  OutDataTypeStr=Inherit: Same as first input
  Mux : Mux  Inputs=3
  gain1 : Constant  Value=p_ki  OutDataTypeStr=single
  gain2 : Constant  Value=q_ki  OutDataTypeStr=single
  gain3 : Constant  Value=r_ki  OutDataTypeStr=single
  i_out : Outport
  wires:
  err/1 -> Multiply/2
  gain2/1 -> Mux/2
  gain1/1 -> Mux/1
  gain3/1 -> Mux/3
  reset/1 -> Discrete-Time Integrator/2
  Constant/1 -> Discrete-Time Integrator/3
  Discrete-Time Integrator/1 -> i_out/1
  Mux/1 -> Multiply/1
  Multiply/1 -> Discrete-Time Integrator/1

== system Controller/Controller/Horizontal_Control/Attitude_Controller/Inner_Loop/Rate_Controller/PID_Controller/P_Control ==
  err : Inport
  Multiply : Product  OutDataTypeStr=Inherit: Same as first input
  Mux : Mux  Inputs=3
  gain1 : Constant  Value=p_kp  OutDataTypeStr=single
  gain2 : Constant  Value=q_kp  OutDataTypeStr=single
  gain3 : Constant  Value=r_kp  OutDataTypeStr=single
  p_out : Outport
  wires:
  err/1 -> Multiply/2
  gain2/1 -> Mux/2
  Mux/1 -> Multiply/1
  gain1/1 -> Mux/1
  Multiply/1 -> p_out/1
  gain3/1 -> Mux/3

== system Controller/Controller/Horizontal_Control/Attitude_Controller/Outter_Loop/Attitude_Controller/Error/Bus_Select ==
  INS_Out : Inport
  Bus Selector1 : BusSelector  OutputSignals=phi,theta
  Mux1 : Mux  Inputs=2
  att_est_B_rad : Outport
  wires:
  Bus Selector1/2 -> Mux1/2  "<theta>"
  Bus Selector1/1 -> Mux1/1  "<phi>"
  Mux1/1 -> att_est_B_rad/1
  INS_Out/1 -> Bus Selector1/1

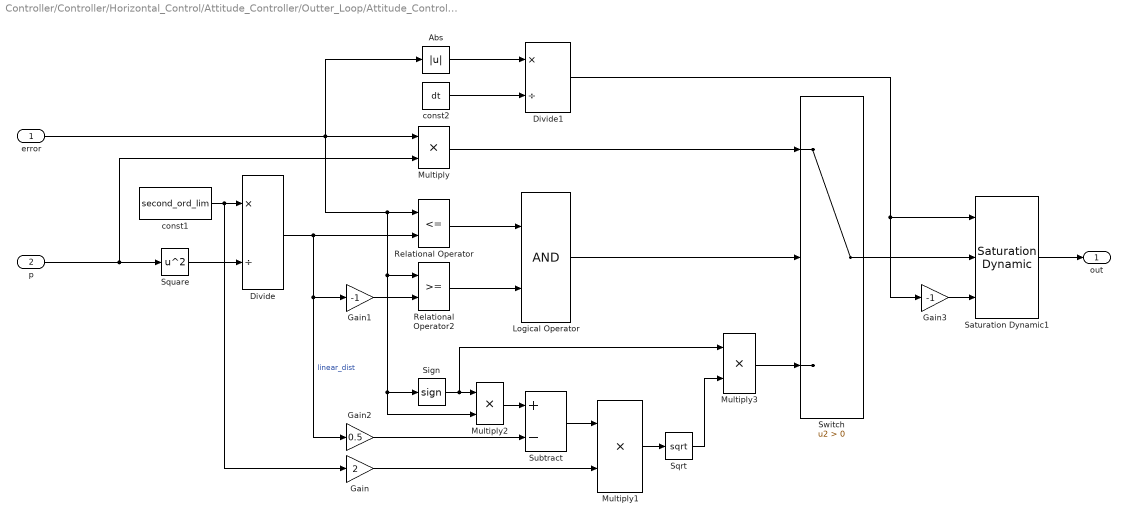
== system Controller/Controller/Horizontal_Control/Attitude_Controller/Outter_Loop/Attitude_Controller/Sqrt_Root_Controller/Sqrt_Root_Control ==
  error : Inport
  p : Inport  Port=2
  Abs : Abs
  Divide : Product  Inputs=*/
  Divide1 : Product  Inputs=*/
  Gain : Gain  Gain=2  OutDataTypeStr=Inherit: Same as input
  Gain1 : Gain  Gain=-1  OutDataTypeStr=Inherit: Same as input
  Gain2 : Gain  Gain=0.5  OutDataTypeStr=Inherit: Same as input
  Gain3 : Gain  Gain=-1  OutDataTypeStr=Inherit: Same as input
  Logical Operator : Logic  AllPortsSameDT=off  OutDataTypeStr=boolean
  Multiply{,1..3} (4 alike) : Product
  Relational Operator : RelationalOperator  Operator=<=  OutDataTypeStr=boolean  RndMeth=Simplest
  Relational Operator2 : RelationalOperator  OutDataTypeStr=boolean  RndMeth=Simplest
  Saturation Dynamic1 : simulink/Discontinuities/Saturation Dynamic  OutMin=[]  OutMax=[]  OutDataTypeStr=Inherit: Same as second input  OutDataType=fixdt(1, 16)  OutScaling=2^-10  DoSatur=off
  Sign : Signum
  Sqrt : Sqrt  SaturateOnIntegerOverflow=on
  Square : Math  Operator=square  SaturateOnIntegerOverflow=on
  Subtract : Sum  Inputs=+-
  Switch : Switch  Criteria=u2 > Threshold
  const1 : Constant  Value=second_ord_lim  OutDataTypeStr=single
  const2 : Constant  Value=dt  OutDataTypeStr=single
  out : Outport
  wires:
  p/1 -> Multiply/2, Square/1
  const1/1 -> Gain/1, Divide/1
  Square/1 -> Divide/2
  Divide/1 -> Gain2/1, Gain1/1, Relational Operator/2  "linear_dist"
  error/1 -> Abs/1, Multiply/1, Multiply2/2, Sign/1, Relational Operator2/1, Relational Operator/1
  Relational Operator/1 -> Logical Operator/1
  Multiply/1 -> Switch/1
  Switch/1 -> Saturation Dynamic1/2
  Multiply3/1 -> Switch/3
  Gain/1 -> Multiply1/2
  Gain1/1 -> Relational Operator2/2
  Relational Operator2/1 -> Logical Operator/2
  Logical Operator/1 -> Switch/2
  Gain2/1 -> Subtract/2
  Sign/1 -> Multiply3/1, Multiply2/1
  Multiply2/1 -> Subtract/1
  Subtract/1 -> Multiply1/1
  Multiply1/1 -> Sqrt/1
  Sqrt/1 -> Multiply3/2
  Saturation Dynamic1/1 -> out/1
  Abs/1 -> Divide1/1
  const2/1 -> Divide1/2
  Divide1/1 -> Gain3/1, Saturation Dynamic1/1
  Gain3/1 -> Saturation Dynamic1/3
